simulink model "SvolgimentoEsame_SIM"  (R2025b)
settings: Solver=VariableStepAuto  StartTime=0.0  StopTime=10.0  RelTol=1e-3
values from neighbouring files (symbols this model uses):
  A = double(subs(A_sym, p_eq_instabile, val_instabili))    [SvolgimentoEsame.m]
  B = double(subs(B_sym, p_eq_instabile, val_instabili))    [SvolgimentoEsame.m]
  C = eye(4)    [SvolgimentoEsame.m]
  D = zeros(4, 1)    [SvolgimentoEsame.m]
  X_initial = [x0; dx0; th0; dth0]    [SvolgimentoEsame.m]
undefined symbols (not defined in the file or in its folder): K
settings Model: Creator=salvo  LastModifiedBy=salvo

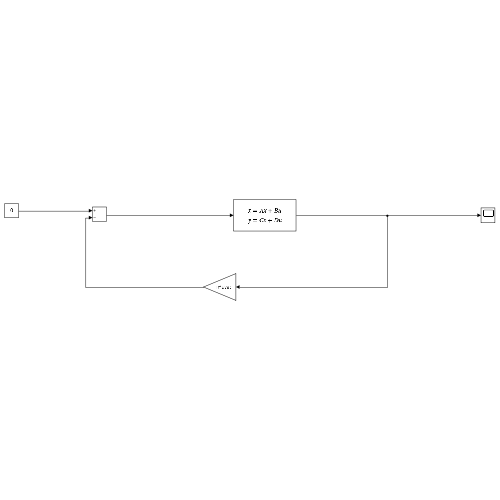
[thumbnail: Simulink's stored preview of the top-level diagram]
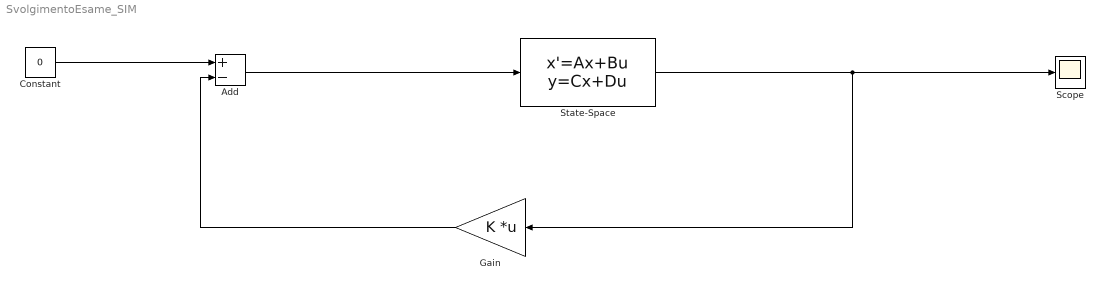
== system SvolgimentoEsame_SIM ==
  Add : Sum  Inputs=+-
  Constant : Constant  Value=0
  Gain : Gain  Gain=K  Multiplication=Matrix(K*u) (u vector)
  Scope : Scope
      settings: ActiveDisplayYMinimum=-2.8870887881109031  ActiveDisplayYMaximum=1.93168681019771
  State-Space : StateSpace  A=A  B=B  C=C  D=D  InitialCondition=X_initial
  wires:
  Gain/1 -> Add/2
  Add/1 -> State-Space/1
  State-Space/1 -> Scope/1, Gain/1
  Constant/1 -> Add/1
